simulink model "SinglephasePVArray"  (R2024a)
settings: Solver=VariableStepAuto  StartTime=0.0  StopTime=2  RelTol=1e-3
undefined symbols (not defined in the file): DiscIntNeverNeededParam
libraries: spsSeriesRLCBranchLib x9, spsCurrentMeasurementLib x4, spsIGBTDiodeLib x4, simulink x2, spsUniversalBridgeLib x2, spsVoltageMeasurementLib x2, spsACVoltageSourceLib x1, spsBreakerLib x1, spsDiodeLib x1, spsGroundLib x1, spsIGBTLib x1, spsPVArrayLib x1
settings Model: Creator=aditl  LastModifiedBy=aditl

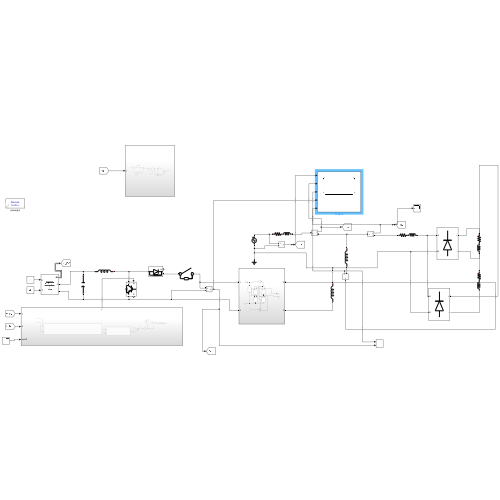
[thumbnail: Simulink's stored preview of the top-level diagram]
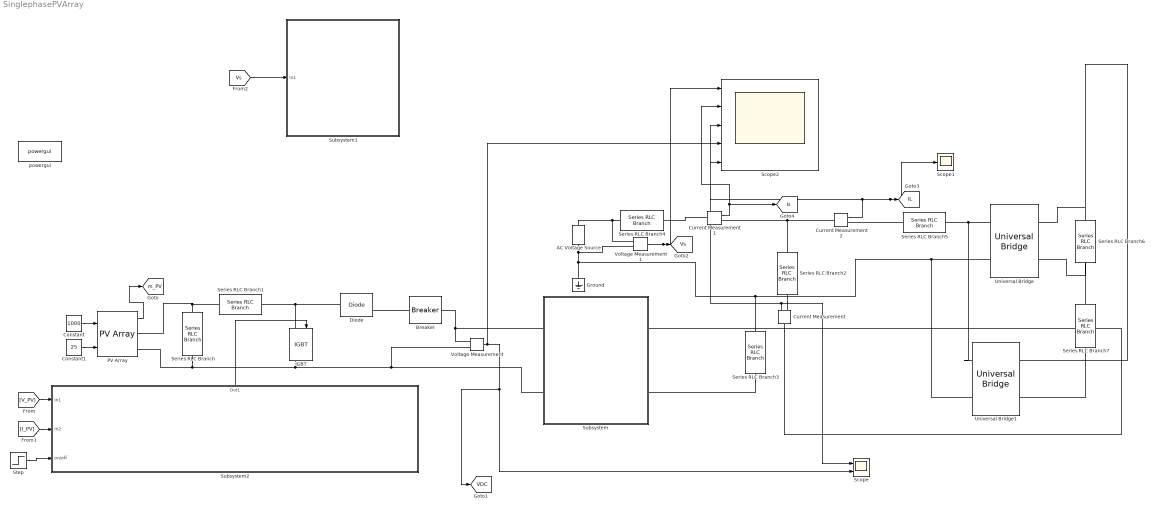
== system SinglephasePVArray ==
  AC Voltage Source : spsACVoltageSourceLib/AC Voltage Source  Amplitude=230  Phase=0  Frequency=50  SampleTime=0  Measurements=None  BusType=swing  Pref=10e3  Qref=0  Qmin=-inf  Qmax=+inf
  Breaker : spsBreakerLib/Breaker  InitialState=0  SwitchingTimes=[0.5]  External=off  BreakerResistance=0.01  SnubberResistance=1e6  SnubberCapacitance=inf  Measurements=None  MoreParameters=on  NoBreakLoop=off
  Constant : Constant  Value=1000
  Constant1 : Constant  Value=25
  Current Measurement : spsCurrentMeasurementLib/Current Measurement  PhasorSimulation=off  OutputType=Complex  PSBequivalent=0
  Current Measurement1 : spsCurrentMeasurementLib/Current Measurement  PhasorSimulation=off  OutputType=Complex  PSBequivalent=0
  Current Measurement2 : spsCurrentMeasurementLib/Current Measurement  PhasorSimulation=off  OutputType=Complex  PSBequivalent=0
  Diode : spsDiodeLib/Diode  Ron=0.001  Lon=0  Vf=0.8  IC=0  UseSnubber=0  Rs=500  Cs=250e-9  Measurements=on
  Ground : spsGroundLib/Ground  LConnTagsString=a
  IGBT : spsIGBTLib/IGBT  Ron=0.001  Lon=0  Vf=1  Tf=1e-6  Tt=2e-6  IC=0  Rs=1e5  Cs=inf  Measurements=on
  PV Array : spsPVArrayLib/PV Array  Npar=1  Nser=5  PlotType=array @ 1000 W/m2 & specified temperatures  S_vec="[ 1000  500  100 ]"  Temp_C_vec="[ 45 25  ]"  ModuleName=Aleo Solar S79y270  PlotWhenSelected=off  Pm=271.61  Ncell=60  Voc=38.6  Isc=9.2  Vm=31.4  Im=8.65  beta_Voc_pc=-0.299  alpha_Isc_pc=0.031  beta_Voc=-0.11541  alpha_Isc=0.002852  IL=9.2483  I0=2.9223e-11  nI=0.94638  Rsh=194.6187  Rs=0.31978  RobustModel=off  RobustCellTemperature=313.3991  BAL=on  Tc=1e-6  Tfilter=5e-5
  Scope : Scope  NumInputPorts=2
  Scope1 : Scope
  Scope2 : Scope  NumInputPorts=5
  Series RLC Branch : spsSeriesRLCBranchLib/Series RLC Branch  LConnTagsString=__new0  RConnTagsString=__new0  BranchType=C  Resistance=1  Inductance=1e-3  SetiL0=off  InitialCurrent=0  Capacitance=100e-6  Setx0=off  InitialVoltage=0  Measurements=None
  Series RLC Branch1 : spsSeriesRLCBranchLib/Series RLC Branch  LConnTagsString=__new0  RConnTagsString=__new0  BranchType=L  Resistance=1  Inductance=4e-3  SetiL0=off  InitialCurrent=0  Capacitance=1e-6  Setx0=off  InitialVoltage=0  Measurements=None
  Series RLC Branch2 : spsSeriesRLCBranchLib/Series RLC Branch  LConnTagsString=__new0  RConnTagsString=__new0  BranchType=L  Resistance=1  Inductance=2e-3  SetiL0=off  InitialCurrent=0  Capacitance=1e-6  Setx0=off  InitialVoltage=0  Measurements=None
  Series RLC Branch3 : spsSeriesRLCBranchLib/Series RLC Branch  LConnTagsString=__new0  RConnTagsString=__new0  BranchType=L  Resistance=1  Inductance=2e-3  SetiL0=off  InitialCurrent=0  Capacitance=1e-6  Setx0=off  InitialVoltage=0  Measurements=None
  Series RLC Branch4 : spsSeriesRLCBranchLib/Series RLC Branch  LConnTagsString=__new0  RConnTagsString=__new0  BranchType=RL  Resistance=0.2  Inductance=1e-3  SetiL0=off  InitialCurrent=0  Capacitance=1e-6  Setx0=off  InitialVoltage=0  Measurements=None
  Series RLC Branch5 : spsSeriesRLCBranchLib/Series RLC Branch  LConnTagsString=__new0  RConnTagsString=__new0  BranchType=RL  Resistance=0.2  Inductance=1e-3  SetiL0=off  InitialCurrent=0  Capacitance=1e-6  Setx0=off  InitialVoltage=0  Measurements=None
  Series RLC Branch6 : spsSeriesRLCBranchLib/Series RLC Branch  LConnTagsString=__new0  RConnTagsString=__new0  BranchType=RL  Resistance=15  Inductance=100e-3  SetiL0=off  InitialCurrent=0  Capacitance=1e-6  Setx0=off  InitialVoltage=0  Measurements=None
  Series RLC Branch7 : spsSeriesRLCBranchLib/Series RLC Branch  LConnTagsString=__new0  RConnTagsString=__new0  BranchType=RL  Resistance=15  Inductance=100e-3  SetiL0=off  InitialCurrent=0  Capacitance=1e-6  Setx0=off  InitialVoltage=0  Measurements=None
  Step : Step  SampleTime=0
  Subsystem : Subsystem
  Subsystem1 : Subsystem
  Subsystem2 : Subsystem
      settings: PortSchema="{\"entries\":[{\"content\":{\"sides\":[{\"content\":{\"connectorIds\":[\"In1\",\"In2\",\"In3\"]},\"type\":\"ConnectorPlacement.EquallySpacedRectSide\",\"uuid\":\"14786eec-0241-4e35-83c3-907b121b9eb2\"},{\"content\":{\"side\":\"RIGHT\"},\"type\":\"ConnectorPlacement.EquallySpacedRectSide\",\"uuid\":\"173d27b1-7f65-4748-b114-d30920d37356\"},{\"content\":{\"connectorIds\":[\"Out1\"],\"side\":\"TOP\"},\"type\":\"ConnectorPlacement.EquallySpacedRectSide\",\"uuid\":\"0281ca9d-ded6-4f23-8408-9b2f869d84fc\"}]},\"type\":\"ConnectorPlacement.EquallySpacedConnector\",\"uuid\":\"7aa841fd-ffaf-4919-a8b6-3c96325493f5\"}],\"packageUris\":[\"http://schema.mathworks.com/mf0/Connector/R2020b\"],\"version\":\"1.0\"}"
  Universal Bridge : spsUniversalBridgeLib/Universal Bridge  Arms=2  SnubberResistance=1e5  SnubberCapacitance=inf  Device=Diodes  Ron=1e-3  Lon=0  ForwardVoltages="[  0  0  ]"  ForwardVoltage=0  GTOparameters=[ 10e-6 , 20e-6 ]  IGBTparameters=[ 1e-6 , 2e-6 ]  Measurements=None  Measurements_2=None  converterType=Rectifier
  Universal Bridge1 : spsUniversalBridgeLib/Universal Bridge  Arms=2  SnubberResistance=1e5  SnubberCapacitance=inf  Device=Diodes  Ron=1e-3  Lon=0  ForwardVoltages="[  0  0  ]"  ForwardVoltage=0  GTOparameters=[ 10e-6 , 20e-6 ]  IGBTparameters=[ 1e-6 , 2e-6 ]  Measurements=None  Measurements_2=None  converterType=Rectifier
  Voltage Measurement : spsVoltageMeasurementLib/Voltage Measurement  PhasorSimulation=off  OutputType=Complex  PSBequivalent=0
  Voltage Measurement1 : spsVoltageMeasurementLib/Voltage Measurement  PhasorSimulation=off  OutputType=Complex  PSBequivalent=0
  powergui : sps_lib/powergui  Priority=1  SimulationMode=Discrete  SampleTime=1e-5  frequency=60  Iterations=50  frequencyindice=50  Pbase=100e6  ErrMax=1e-4  UnitsV=kV  UnitsW=MW  buscounter=0  FunctionMessages=off  echomessages=off  EnableUseOfTLC=off  CurrentSourceSwitches=off  DisableSnubberDevices=off  DisableRonSwitches=off  DisableVfSwitches=off  DisplayEquations=off  AutomaticDiscreteSolvers=off  SolverType=Tustin/Backward Euler (TBE)  Interpol=off  ExternalGateDelay=off  methode=off  Ts=100  x0status=blocks  SPID=on  SwTol=0  HookPort=off  NonlinearTolerance=1e-4  nMaxIteration=100  ContinueOnMaxIteration=off  RestoreLinks=warning  ResistiveCurrentMeasurement=off  Frange=[0:2:500]  Ylog=off  Xlog=on  ShowGrid=off  save=off  variable=ZData  structure=0  ZoomFFT=off  StartTime=0.0  cycles=1  DisplayStyle=1  fundamental=60  FreqAxis=off  MaxFrequency=1000  frequencyindicesteady=1  RmsSteady=1  display=off
  tag scope: IL=global, Is=global, VDC=global, Vs=global, m_PV=global
  wires:
  Constant/1 -> PV Array/1
  Constant1/1 -> PV Array/2
  PV Array/1 -> [m_PV]
  [V_PV] -> Subsystem2/1(In1)
  [I_PV] -> Subsystem2/2(In2)
  Subsystem2/1(Out1) -> IGBT/1
  Step/1 -> Subsystem2/3(on/off)
  Current Measurement/1 -> Scope/1, Scope2/5
  Voltage Measurement/1 -> Scope2/4, [VDC], Scope/2
  Voltage Measurement1/1 -> Scope2/1, [Vs]
  Current Measurement2/1 -> Scope1/1, [IL], Scope2/3
  Current Measurement1/1 -> [Is], Scope2/2
  [Vs] -> Subsystem1/1(In1)
  connections:
  Series RLC Branch/LConn1 -- Series RLC Branch1/RConn1 -- PV Array/RConn1
  Series RLC Branch/RConn1 -- Voltage Measurement/LConn2 -- Subsystem/LConn2 -- IGBT/RConn1 -- PV Array/RConn2
  IGBT/LConn1 -- Diode/LConn1 -- Series RLC Branch1/LConn1
  Breaker/LConn1 -- Diode/RConn1
  Voltage Measurement/LConn1 -- Subsystem/LConn1 -- Breaker/RConn1
  Current Measurement/LConn1 -- Subsystem/RConn1
  Series RLC Branch2/RConn1 -- Current Measurement/RConn1
  Series RLC Branch3/RConn1 -- Subsystem/RConn2
  Series RLC Branch4/LConn1 -- AC Voltage Source/RConn1 -- Voltage Measurement1/LConn1
  Ground/LConn1 -- Universal Bridge1/LConn2 -- Universal Bridge/LConn2 -- Series RLC Branch3/LConn1 -- Voltage Measurement1/LConn2 -- AC Voltage Source/LConn1
  Current Measurement1/LConn1 -- Series RLC Branch4/RConn1
  Current Measurement2/LConn1 -- Current Measurement1/RConn1 -- Series RLC Branch2/LConn1
  Series RLC Branch5/LConn1 -- Current Measurement2/RConn1
  Universal Bridge/LConn1 -- Universal Bridge1/LConn1 -- Series RLC Branch5/RConn1
  Series RLC Branch6/LConn1 -- Universal Bridge/RConn1
  Series RLC Branch6/RConn1 -- Universal Bridge/RConn2
  Series RLC Branch7/LConn1 -- Universal Bridge1/RConn1
  Series RLC Branch7/RConn1 -- Universal Bridge1/RConn2

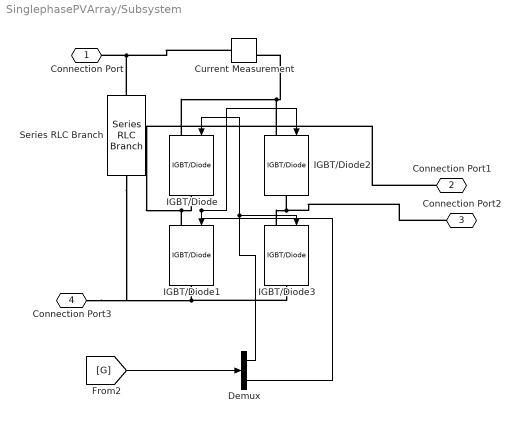
== system SinglephasePVArray/Subsystem ==
  Current Measurement : spsCurrentMeasurementLib/Current Measurement  PhasorSimulation=off  OutputType=Complex  PSBequivalent=0
  Demux : Demux  Outputs=2
  IGBT/Diode{,1..3} (4 alike) : spsIGBTDiodeLib/IGBT//Diode  Ron=1e-3  Rs=1e5  Cs=inf  Measurements=off
  Series RLC Branch : spsSeriesRLCBranchLib/Series RLC Branch  LConnTagsString=__new0  RConnTagsString=__new0  BranchType=C  Resistance=1  Inductance=1e-3  SetiL0=off  InitialCurrent=0  Capacitance=1500e-6  Setx0=on  InitialVoltage=350  Measurements=None
  Connection Port : PMIOPort  Side=Left
  Connection Port1 : PMIOPort  Port=2  Side=Right
  Connection Port2 : PMIOPort  Port=3  Side=Right
  Connection Port3 : PMIOPort  Port=4  Side=Left
  wires:
  [G] -> Demux/1
  Demux/2 -> IGBT/Diode2/1, IGBT/Diode1/1
  Demux/1 -> IGBT/Diode/1, IGBT/Diode3/1
  connections:
  IGBT/Diode1/LConn1 -- Connection Port1/RConn1 -- IGBT/Diode/RConn1
  IGBT/Diode/LConn1 -- IGBT/Diode2/LConn1 -- Current Measurement/RConn1
  IGBT/Diode3/RConn1 -- Connection Port3/RConn1 -- Series RLC Branch/RConn1 -- IGBT/Diode1/RConn1
  IGBT/Diode3/LConn1 -- Connection Port2/RConn1 -- IGBT/Diode2/RConn1
  Current Measurement/LConn1 -- Series RLC Branch/LConn1 -- Connection Port/RConn1

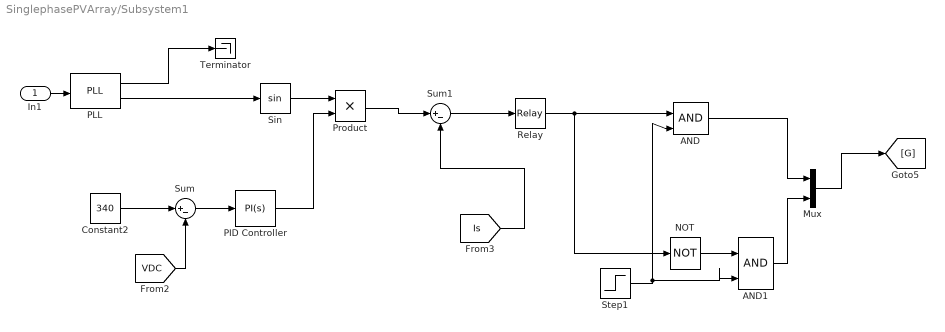
== system SinglephasePVArray/Subsystem1 ==
  In1 : Inport
  AND : Logic  IconShape=distinctive  AllPortsSameDT=off  OutDataTypeStr=boolean
  AND1 : Logic  IconShape=distinctive  AllPortsSameDT=off  OutDataTypeStr=boolean
  Constant2 : Constant  Value=340
  Mux : Mux  Inputs=2
  NOT : Logic  Operator=NOT  IconShape=distinctive  AllPortsSameDT=off  OutDataTypeStr=boolean
  PID Controller : slpidlib/PID Controller  Controller=PI  Form=Parallel  TimeDomain=Continuous-time  UseExternalTs=off  SampleTime=-1  IntegratorMethod=Forward Euler  FilterMethod=Forward Euler  ControllerParametersSource=internal  P=1  I=1  UseKiTs=off  D=0  UseExternalDerivativeSource=off  N=100  UseFilter=on  TunerSelectOption=Transfer Function Based (PID Tuner App)  InitialConditionSource=internal  InitialConditionForIntegrator=0  InitialConditionForFilter=0  DifferentiatorICPrevScaledInput=0  ExternalReset=none  TrackingMode=off  Kt=1  LimitOutput=off  SatLimitsSource=internal  UpperSaturationLimit=inf  LowerSaturationLimit=-inf  LinearizeAsGain=on  AntiWindupMode=none  Kb=1  LimitIntegrator=off  UpperIntegratorSaturationLimit=inf  LowerIntegratorSaturationLimit=-inf  POutMin=[]  POutMax=[]  IOutMin=[]  IOutMax=[]  DOutMin=[]  DOutMax=[]  NOutMin=[]  NOutMax=[]  SumOutMin=[]  SumOutMax=[]  SaturationOutMin=[]  SaturationOutMax=[]  PParamMin=[]  PParamMax=[]  IParamMin=[]  IParamMax=[]  DParamMin=[]  DParamMax=[]  NParamMin=[]  NParamMax=[]  KbParamMin=[]  KbParamMax=[]  KtParamMin=[]  KtParamMax=[]  KbOutMin=[]  KbOutMax=[]  KtOutMin=[]  KtOutMax=[]  IntegratorOutMin=[]  IntegratorOutMax=[]  FilterOutMin=[]  FilterOutMax=[]  SumI1OutMin=[]  SumI1OutMax=[]  SumI2OutMin=[]  SumI2OutMax=[]  SumI3OutMin=[]  SumI3OutMax=[]  SumI4OutMin=[]  SumI4OutMax=[]  SumDOutMin=[]  SumDOutMax=[]  DifferentiatorOutMin=[]  DifferentiatorOutMax=[]  FilterDiffOutCoefMin=[]  FilterDiffOutCoefMax=[]  ReciprocalOutMin=[]  ReciprocalOutMax=[]  SumDenOutMin=[]  SumDenOutMax=[]  SumNumOutMin=[]  SumNumOutMax=[]  DivideOutMin=[]  DivideOutMax=[]  UdiffTsProdOutMin=[]  UdiffTsProdOutMax=[]  NTsProdOutMin=[]  NTsProdOutMax=[]  UintegralTsProdOutMin=[]  UintegralTsProdOutMax=[]  UngainTsProdOutMin=[]  UngainTsProdOutMax=[]  ClampingZeroOutDataTypeStr=Inherit: Inherit via back propagation  ClampingZeroOutMin=[]  ClampingZeroOutMax=[]  FilterDenConstantOutDataTypeStr=Inherit: Inherit via back propagation  FilterDenConstantOutMin=[]  FilterDenConstantOutMax=[]  PCopyOutDataTypeStr=Inherit: Inherit via back propagation  PCopyOutMin=[]  PCopyOutMax=[]  NCopyOutDataTypeStr=Inherit: Inherit via back propagation  NCopyOutMin=[]  NCopyOutMax=[]  IntegratorContinuousStateAttributes=''  IntegratorStateMustResolveToSignalObject=off  IntegratorRTWStateStorageClass=Auto  FilterContinuousStateAttributes=''  FilterStateMustResolveToSignalObject=off  FilterRTWStateStorageClass=Auto  ParallelPVariant=InternalParameters  IdealPVariant=Disabled  IVariant=InternalParameters  DVariant=Disabled  IntegratorVariant=Continuous  SatVariant=Disabled  AWVariant=Passthrough  PCopyVariant=Disabled  TRVariant=Disabled  FdbkBlocksVariant=Forward  IdealPFdbkVariant=Disabled  SatFdbkVariant=Disabled  DerivativeFilterVariant=Disabled  NVariant=Disabled  NCopyVariant=Disabled_SignalSpec  FilterICVariant=Disabled  IntegratorICVariant=InternalICs  ExternalResetVariant=Disabled  TRSumVariant=Passthrough  SumFdbkVariant=Disabled  SumVariant=Sum_PI  TsampFilterVariant=InternalTs  TsampNgainVariant=Passthrough  TsampIntegralVariant=Disabled_SignalSpec  ExternalSaturationOutDataTypeStr=Inherit: Same as second input  DerivativeSourceVariant=Disabled
  PLL : spsPLLLib/PLL  Fmin=45  Par_Init=[0, 60]  ParK=[180, 3200, 1]  TcD=1e-4  MaxRateChangeFreq=12  FilterCutOffFreq=25  Ts=0  AGC=on
      settings: LibrarySourceBlock=sps_lib/Control/PLL
  Product : Product
  Relay : Relay  OnSwitchValue=0.02  OffSwitchValue=-0.02
  Sin : Trigonometry
  Step1 : Step  SampleTime=0
  Sum : Sum  Inputs=|+-
  Sum1 : Sum  Inputs=|+-
  Terminator : Terminator
  wires:
  PID Controller/1 -> Product/2
  AND1/1 -> Mux/2
  PLL/2 -> Sin/1
  Mux/1 -> [G]
  Sum1/1 -> Relay/1
  AND/1 -> Mux/1
  [Is] -> Sum1/2
  In1/1 -> PLL/1
  Step1/1 -> AND1/2, AND/2
  PLL/1 -> Terminator/1
  NOT/1 -> AND1/1
  Product/1 -> Sum1/1
  Sin/1 -> Product/1
  Sum/1 -> PID Controller/1
  Relay/1 -> NOT/1, AND/1
  [VDC] -> Sum/2
  Constant2/1 -> Sum/1

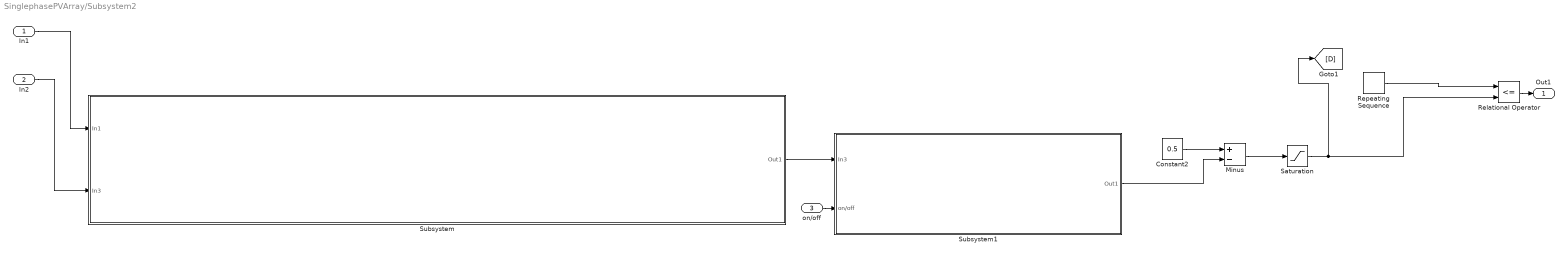
== system SinglephasePVArray/Subsystem2 ==
  In1 : Inport
  In2 : Inport  Port=2
  on/off : Inport  Port=3
  Constant2 : Constant  Value=0.5
  Minus : Sum  Inputs=+-
  Relational Operator : RelationalOperator  Operator=<=  OutDataTypeStr=boolean  RndMeth=Simplest  InputSameDT=off
  Repeating Sequence : simulink/Sources/Repeating Sequence  rep_seq_t=[0 1/5000]  rep_seq_y=[0 1]
  Saturation : Saturate  UpperLimit=0.99  LowerLimit=0.01
  Subsystem : Subsystem
  Subsystem1 : Subsystem
  Out1 : Outport
  wires:
  Subsystem1/1(Out1) -> Minus/2
  Saturation/1 -> [D], Relational Operator/2
  Minus/1 -> Saturation/1
  Subsystem/1(Out1) -> Subsystem1/1(In3)
  Relational Operator/1 -> Out1/1
  Repeating Sequence/1 -> Relational Operator/1
  Constant2/1 -> Minus/1
  on/off/1 -> Subsystem1/2(on/off)
  In2/1 -> Subsystem/2(In3)
  In1/1 -> Subsystem/1(In1)

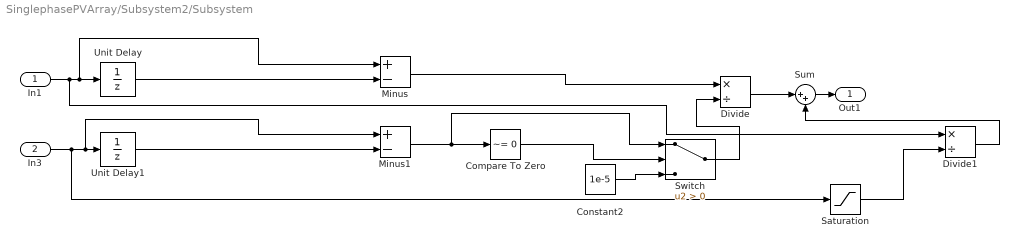
== system SinglephasePVArray/Subsystem2/Subsystem ==
  In1 : Inport
  In3 : Inport  Port=2
  Compare To Zero : simulink/Logic and Bit Operations/Compare To Zero  relop=~=  OutDataTypeStr=boolean
  Constant2 : Constant  Value=1e-5
  Divide : Product  Inputs=*/
  Divide1 : Product  Inputs=*/
  Minus : Sum  Inputs=+-
  Minus1 : Sum  Inputs=+-
  Saturation : Saturate  UpperLimit=inf  LowerLimit=eps
  Sum : Sum  Inputs=|++
  Switch : Switch  Criteria=u2 > Threshold  SaturateOnIntegerOverflow=off  InputSameDT=off
  Unit Delay : UnitDelay  SampleTime=-1  HasFrameUpgradeWarning=on
  Unit Delay1 : UnitDelay  SampleTime=-1  HasFrameUpgradeWarning=on
  Out1 : Outport
  wires:
  Sum/1 -> Out1/1
  Unit Delay/1 -> Minus/2
  In1/1 -> Divide1/1, Minus/1, Unit Delay/1
  Unit Delay1/1 -> Minus1/2
  Divide1/1 -> Sum/2
  Constant2/1 -> Switch/3
  Saturation/1 -> Divide1/2
  Minus/1 -> Divide/1
  Divide/1 -> Sum/1
  Compare To Zero/1 -> Switch/2
  Minus1/1 -> Switch/1, Compare To Zero/1
  Switch/1 -> Divide/2
  In3/1 -> Saturation/1, Minus1/1, Unit Delay1/1

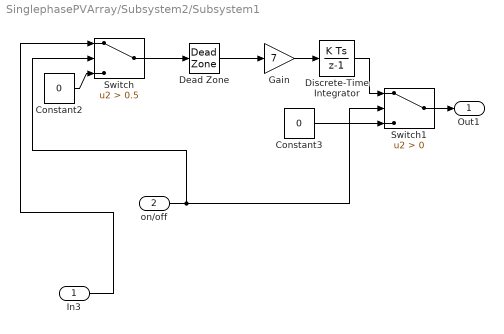
== system SinglephasePVArray/Subsystem2/Subsystem1 ==
  In3 : Inport
  on/off : Inport  Port=2
  Constant2 : Constant  Value=0
  Constant3 : Constant  Value=0
  Dead Zone : DeadZone  LowerValue=-0.06  UpperValue=0.06
  Discrete-Time Integrator : DiscreteIntegrator  gainval=1.8  SampleTime=1e-5  LimitOutput=on  UpperSaturationLimit=1  LowerSaturationLimit=-1  ICPrevOutput=DiscIntNeverNeededParam  ICPrevScaledInput=DiscIntNeverNeededParam
  Gain : Gain  Gain=7
  Switch : Switch  Criteria=u2 > Threshold  Threshold=0.5  SaturateOnIntegerOverflow=off  InputSameDT=off
  Switch1 : Switch  Criteria=u2 > Threshold  SaturateOnIntegerOverflow=off  InputSameDT=off
  Out1 : Outport
  wires:
  Discrete-Time Integrator/1 -> Switch1/1
  Constant2/1 -> Switch/3
  on/off/1 -> Switch/2, Switch1/2
  Switch/1 -> Dead Zone/1
  Gain/1 -> Discrete-Time Integrator/1
  Constant3/1 -> Switch1/3
  Dead Zone/1 -> Gain/1
  Switch1/1 -> Out1/1
  In3/1 -> Switch/1
